simulink library "rotation_visualization_lib"  (R2016b)
settings: Solver=VariableStepAuto  StartTime=0.0  StopTime=10.0  RelTol=1e-3
settings Model: Creator=Sean  LastModifiedBy=Sean

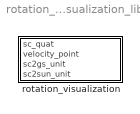
== system rotation_visualization_lib ==
  rotation_visualization : Subsystem

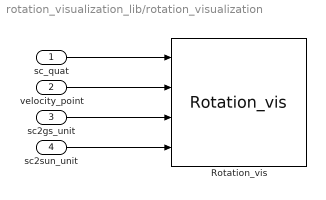
== system rotation_visualization_lib/rotation_visualization ==
  sc_quat : Inport
  velocity_point : Inport  Port=2
  sc2gs_unit : Inport  Port=3
  sc2sun_unit : Inport  Port=4
  Rotation_vis : M-S-Function  FunctionName=Rotation_vis
  wires:
  velocity_point/1 -> Rotation_vis/2
  sc_quat/1 -> Rotation_vis/1
  sc2gs_unit/1 -> Rotation_vis/3
  sc2sun_unit/1 -> Rotation_vis/4
